simulink model "Crazyflie_LQ_control"  (R2020b)
settings: Solver=VariableStepAuto  StartTime=0.0  StopTime=20  RelTol=1e-3
values from neighbouring files (symbols this model uses):
  LQRK = lqr(stateA, stateB, Q, R, N)    [Crazyflie_get_LQ_Gain.m]
  stateA = [0  0  0  1  0  0  0  0  0  0  0  0 ... (first row only)    [Crazyflie_get_LQ_Gain.m]
  stateB = [0   0      0     0 ... (first row only)    [Crazyflie_get_LQ_Gain.m]
  stateC = eye(12)    [Crazyflie_get_LQ_Gain.m]
  stateD = zeros(12, 4)    [Crazyflie_get_LQ_Gain.m]
settings Model: Creator=kt012  LastModifiedBy=kt012

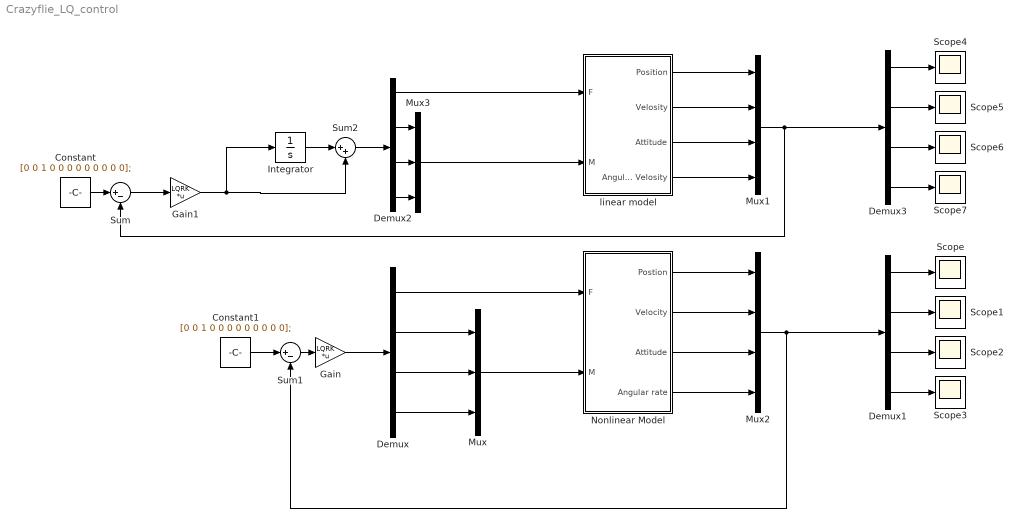
== system Crazyflie_LQ_control ==
  Constant : Constant  Value=[0 0 1 0 0 0 0 0 0 0 0 0];
  Constant1 : Constant  Value=[0 0 1 0 0 0 0 0 0 0 0 0];
  Demux{,1..3} (4 alike) : Demux
  Gain : Gain  Gain=LQRK  Multiplication=Matrix(K*u)
  Gain1 : Gain  Gain=LQRK  Multiplication=Matrix(K*u)
  Integrator : Integrator  InitialCondition=[0 0 0 0]'
  Mux : Mux  Inputs=3
  Mux1 : Mux
  Mux2 : Mux
  Mux3 : Mux  Inputs=3
  Nonlinear Model : Subsystem
  Scope{,1..7} (8 alike) : Scope
  Sum : Sum  Inputs=|+-
  Sum1 : Sum  Inputs=|+-
  Sum2 : Sum  Inputs=|++
  linear model : Subsystem
  wires:
  linear model/3(Attitude) -> Mux1/3
  Demux/1 -> Nonlinear Model/1(F)
  linear model/2(Velosity) -> Mux1/2
  linear model/1(Position) -> Mux1/1
  linear model/4(Angular Velosity) -> Mux1/4
  Mux/1 -> Nonlinear Model/2(M)
  Gain/1 -> Demux/1
  Demux/2 -> Mux/1
  Demux/3 -> Mux/2
  Demux/4 -> Mux/3
  Demux1/1 -> Scope/1
  Demux1/2 -> Scope1/1
  Demux1/3 -> Scope2/1
  Demux1/4 -> Scope3/1
  Nonlinear Model/4(Angular rate) -> Mux2/4
  Nonlinear Model/1(Postion) -> Mux2/1
  Nonlinear Model/2(Velocity) -> Mux2/2
  Nonlinear Model/3(Attitude) -> Mux2/3
  Mux2/1 -> Sum1/2, Demux1/1
  Demux2/4 -> Mux3/3
  Demux2/3 -> Mux3/2
  Demux2/2 -> Mux3/1
  Gain1/1 -> Integrator/1, Sum2/2
  Mux3/1 -> linear model/2(M)
  Demux2/1 -> linear model/1(F)
  Mux1/1 -> Sum/2, Demux3/1
  Demux3/4 -> Scope7/1
  Demux3/3 -> Scope6/1
  Demux3/2 -> Scope5/1
  Demux3/1 -> Scope4/1
  Sum/1 -> Gain1/1
  Constant/1 -> Sum/1
  Constant1/1 -> Sum1/1
  Sum1/1 -> Gain/1
  Integrator/1 -> Sum2/1
  Sum2/1 -> Demux2/1

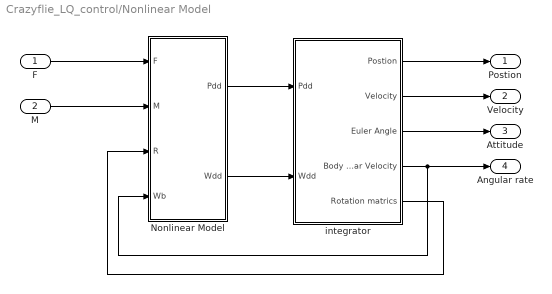
== system Crazyflie_LQ_control/Nonlinear Model ==
  F : Inport
  M : Inport  Port=2
  Nonlinear Model : MATLAB Function  TreatAsAtomicUnit=on
  integrator : Subsystem
  Postion : Outport
  Velocity : Outport  Port=2
  Attitude : Outport  Port=3
  Angular rate : Outport  Port=4
  wires:
  integrator/4(Body Angular Velocity) -> Nonlinear Model/4(Wb), Angular rate/1
  integrator/3(Euler Angle) -> Attitude/1
  Nonlinear Model/1(Pdd) -> integrator/1(Pdd)
  Nonlinear Model/2(Wdd) -> integrator/2(Wdd)
  integrator/2(Velocity) -> Velocity/1
  M/1 -> Nonlinear Model/2(M)
  integrator/1(Postion) -> Postion/1
  F/1 -> Nonlinear Model/1(F)
  integrator/5(Rotation matrics) -> Nonlinear Model/3(R)

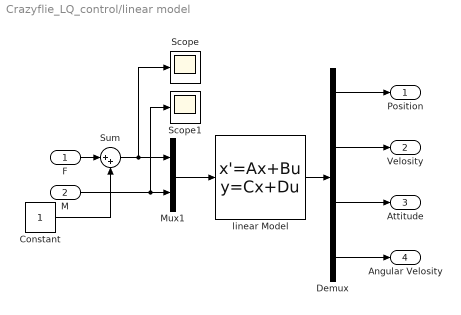
== system Crazyflie_LQ_control/linear model ==
  F : Inport
  M : Inport  Port=2
  Constant : Constant
  Demux : Demux
  Mux1 : Mux  Inputs=2
  Scope : Scope
  Scope1 : Scope
  Sum : Sum  Inputs=|++
  linear Model : StateSpace  A=stateA  B=stateB  C=stateC  D=stateD  InitialCondition=[0 0 0 0 0 0 0 0 0 0 0 0];
  Position : Outport
  Velosity : Outport  Port=2
  Attitude : Outport  Port=3
  Angular Velosity : Outport  Port=4
  wires:
  linear Model/1 -> Demux/1
  Mux1/1 -> linear Model/1
  F/1 -> Sum/1
  Demux/2 -> Velosity/1
  Demux/1 -> Position/1
  Demux/3 -> Attitude/1
  M/1 -> Scope1/1, Mux1/2
  Demux/4 -> Angular Velosity/1
  Constant/1 -> Sum/2
  Sum/1 -> Scope/1, Mux1/1

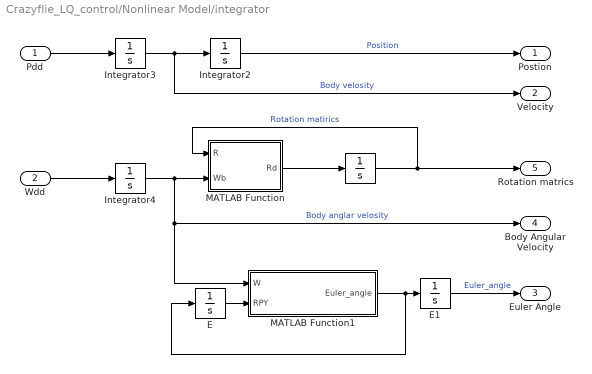
== system Crazyflie_LQ_control/Nonlinear Model/integrator ==
  Pdd : Inport
  Wdd : Inport  Port=2
  " " : Integrator  InitialCondition=[1 0 0; 0 1 0; 0 0 1];  ContinuousStateAttributes="\"\""
  E : Integrator  InitialCondition=[0 0 0];
  E1 : Integrator  InitialCondition=[0 0 0];
  Integrator2 : Integrator  InitialCondition=[0 0.5 0];
  Integrator3 : Integrator  InitialCondition=[0 0 0.0];
  Integrator4 : Integrator  InitialCondition=[0 0 0];  ContinuousStateAttributes='Body_anglar_velocity'
  MATLAB Function : MATLAB Function  TreatAsAtomicUnit=on
  MATLAB Function1 : MATLAB Function  TreatAsAtomicUnit=on
  Postion : Outport
  Velocity : Outport  Port=2
  Euler Angle : Outport  Port=3
  Body Angular Velocity : Outport  Port=4
  Rotation matrics : Outport  Port=5
  wires:
  Integrator4/1 -> Body Angular Velocity/1, MATLAB Function1/1(W), MATLAB Function/2(Wb)  "Body anglar velosity"
  Pdd/1 -> Integrator3/1
  Integrator3/1 -> Integrator2/1, Velocity/1  "Body velosity"
  Integrator2/1 -> Postion/1  "Position"
  Wdd/1 -> Integrator4/1
  " "/1 -> MATLAB Function/1(R), Rotation matrics/1  "Rotation matirics"
  MATLAB Function/1(Rd) -> " "/1
  E/1 -> MATLAB Function1/2(RPY)
  MATLAB Function1/1(Euler_angle) -> E/1, E1/1
  E1/1 -> Euler Angle/1  "Euler_angle"

== matlab function Crazyflie_LQ_control/Nonlinear Model/Nonlinear Model ==
  data: Pdd output; F input; M input; R input; Wb input; Wdd output
function [Pdd,Wdd] = fcn(F, M, R, Wb)
m = 0.027;
e3 = [0 0 1]';
g = 9.8;
% % crazyflie
I = [16.571710 0.830806 0.718277;
     0.830806 16.655602 1.800197;
     0.718277 1.800197 29.261652] * 10^(-6);      % crazyflieの慣性モーメント（kg・m^2）
% I = [1 0 0;
%      0 1 0;
%      0 0 1] * 10^(-6);
% 機体上向き加速度
Pdd = (R*F*e3 - m*g*e3)/m;

% 各加速度計算（ボディー座標系）
Wdd = pinv(I)*(M - cross(Wb, I * Wb));

== matlab function Crazyflie_LQ_control/Nonlinear Model/integrator/MATLAB Function1 ==
  data: W input; Euler_angle output; RPY input
function Euler_angle = fcn(W, RPY)
roll = RPY(1);
pitch = RPY(2);
yaw = RPY(3);
rollS = sin(roll); rollC = cos(roll);           
pitchS = sin(pitch); pitchC = cos(pitch);       


Euler_angle = pinv([1 0 -pitchS;
     0 rollC  pitchC * rollS;
     0 -rollS pitchC * rollC]) * W;

== matlab function Crazyflie_LQ_control/Nonlinear Model/integrator/MATLAB Function ==
  data: R input; Rd output; Wb input
function Rd = fcn(R, Wb)
wx = Wb(1);
wy = Wb(2);
wz = Wb(3);
Wb = [ 0    -wz   wy;
       wz    0   -wx;
      -wy    wx   0];
Rd = R * Wb;
